simulink model "rapid_iv"  (R2024b)
settings: Solver=VariableStepAuto  StartTime=0.0  StopTime=500  RelTol=1e-3
settings Model: Creator=sunzi  LastModifiedBy=sunzi

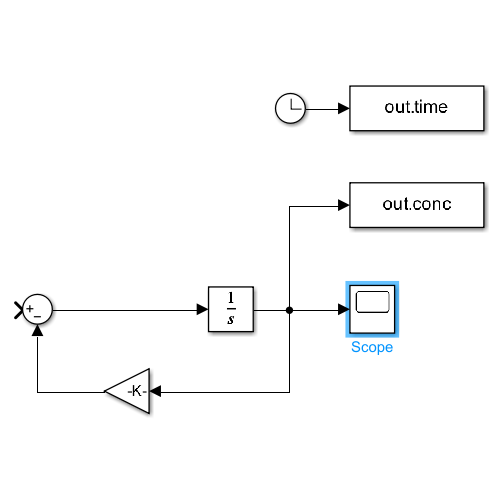
[thumbnail: Simulink's stored preview of the top-level diagram]
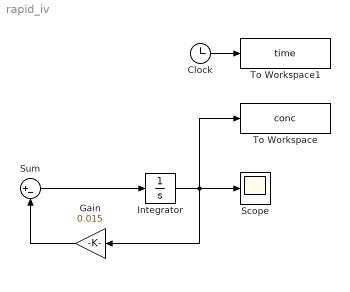
== system rapid_iv ==
  Clock : Clock
  Gain : Gain  Gain=0.015
  Integrator : Integrator  InitialCondition=40/8000
  Scope : Scope
  Sum : Sum  Inputs=|+-
  To Workspace : ToWorkspace  VariableName=conc  SampleTime=-1
  To Workspace1 : ToWorkspace  VariableName=time  SaveFormat=Timeseries  SampleTime=-1
  wires:
  Clock/1 -> To Workspace1/1
  Sum/1 -> Integrator/1
  Gain/1 -> Sum/2
  Integrator/1 -> To Workspace/1, Scope/1, Gain/1
